simulink library "battery_monitor_lib"  (R2022b)
settings: Solver=VariableStepAuto  StartTime=0.0  StopTime=10.0  RelTol=1e-3
settings Model: Creator=dr_pa  LastModifiedBy=LinF

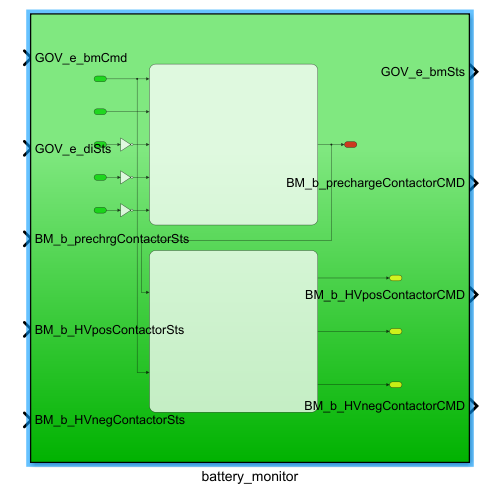
[thumbnail: Simulink's stored preview of the top-level diagram]
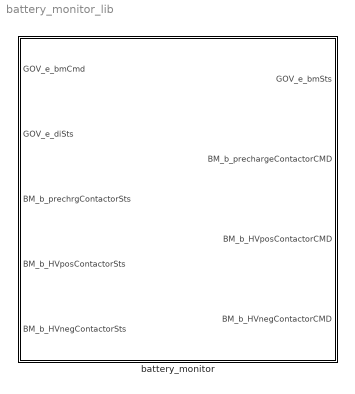
== system battery_monitor_lib ==
  battery_monitor : Subsystem
      settings: LibrarySourceBlock=battery_monitor_lib/battery_monitor

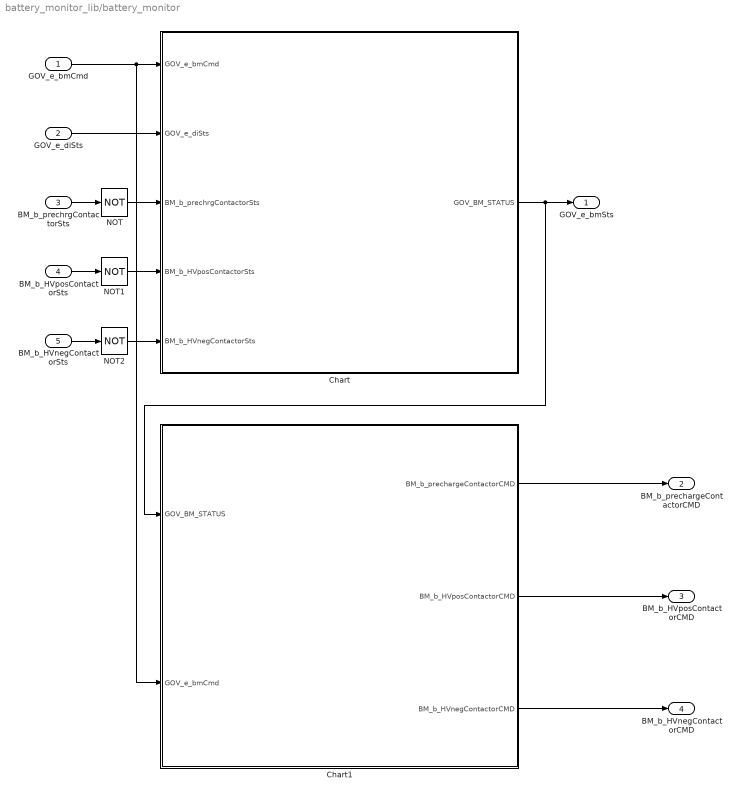
== system battery_monitor_lib/battery_monitor ==
  GOV_e_bmCmd : Inport
  GOV_e_diSts : Inport  Port=2
  BM_b_prechrgContactorSts : Inport  Port=3
  BM_b_HVposContactorSts : Inport  Port=4
  BM_b_HVnegContactorSts : Inport  Port=5
  Chart : Stateflow chart  TreatAsAtomicUnit=on
  Chart1 : Stateflow chart  TreatAsAtomicUnit=on
  NOT : Logic  Operator=NOT  IconShape=distinctive  AllPortsSameDT=off  OutDataTypeStr=boolean
  NOT1 : Logic  Operator=NOT  IconShape=distinctive  AllPortsSameDT=off  OutDataTypeStr=boolean
  NOT2 : Logic  Operator=NOT  IconShape=distinctive  AllPortsSameDT=off  OutDataTypeStr=boolean
  GOV_e_bmSts : Outport
  BM_b_prechargeContactorCMD : Outport  Port=2
  BM_b_HVposContactorCMD : Outport  Port=3
  BM_b_HVnegContactorCMD : Outport  Port=4
  wires:
  GOV_e_bmCmd/1 -> Chart/1(GOV_e_bmCmd), Chart1/2(GOV_e_bmCmd)
  BM_b_prechrgContactorSts/1 -> NOT/1
  BM_b_HVposContactorSts/1 -> NOT1/1
  BM_b_HVnegContactorSts/1 -> NOT2/1
  Chart/1(GOV_BM_STATUS) -> Chart1/1(GOV_BM_STATUS), GOV_e_bmSts/1
  Chart1/2(BM_b_HVposContactorCMD) -> BM_b_HVposContactorCMD/1
  Chart1/1(BM_b_prechargeContactorCMD) -> BM_b_prechargeContactorCMD/1
  Chart1/3(BM_b_HVnegContactorCMD) -> BM_b_HVnegContactorCMD/1
  GOV_e_diSts/1 -> Chart/2(GOV_e_diSts)
  NOT/1 -> Chart/3(BM_b_prechrgContactorSts)
  NOT1/1 -> Chart/4(BM_b_HVposContactorSts)
  NOT2/1 -> Chart/5(BM_b_HVnegContactorSts)

== stateflow chart battery_monitor_lib/battery_monitor/Chart ==
  state ErrorPrechargeClosedState [commented out]
    entry:
    GOV_BM_STATUS = ERR_PRECHARGE_CLOSED;
  state InitialState
    entry:
    GOV_BM_STATUS = BM_INIT;
  state ErrorStartupState
    entry:
    GOV_BM_STATUS = ERR_STARTUP;
  state ErrorAllClosedState [commented out]
    entry:
    GOV_BM_STATUS = ERR_ALL_CLOSED;
  state ErrorHVPositive [commented out]
    entry:
    GOV_BM_STATUS = ERR_HV_POSITIVE;
  state StartupState1
    entry:
    GOV_BM_STATUS = BM_IDLE;
  state StartupState
    entry:
    GOV_BM_STATUS = BM_STARTUP;
  state InitializePrechargeState
    entry:
    GOV_BM_STATUS = INIT_PRECHARGE;
  state ErrorInitializePrechargeState [commented out]
    entry:
    GOV_BM_STATUS = ERR_INIT_PRECHARGE;
  state PrechargeState
    entry:
    GOV_BM_STATUS = PRECHARGE;
  state ErrorPrechargeState [commented out]
    entry:
    GOV_BM_STATUS = ERR_PRECHARGE;
  state RunningState
    entry:
    GOV_BM_STATUS = BM_RUNNING;
  (default) -> InitialState
  InitialState -> ErrorStartupState [order 1] : [BM_b_prechrgContactorSts == 1 && BM_b_HVnegContactorSts == 0 && BM_b_HVposContactorSts == 0]
  InitialState -> ErrorStartupState [order 2] : [BM_b_prechrgContactorSts == 1 && BM_b_HVnegContactorSts == 1 && BM_b_HVposContactorSts == 1]
  InitialState -> ErrorStartupState [order 3] : [BM_b_prechrgContactorSts == 0 && BM_b_HVnegContactorSts == 0 && BM_b_HVposContactorSts == 1]
  RunningState -> InitialState [order 1] : [GOV_e_bmCmd == 1]
  InitialState -> StartupState1 [order 4] : [BM_b_prechrgContactorSts == 0 && BM_b_HVnegContactorSts == 0 && BM_b_HVposContactorSts == 0 && GOV_e_diSts == DI_STATUSES.DRV_START_REQ]
  StartupState -> ErrorStartupState [order 2] : after(100,sec)
  PrechargeState -> ErrorStartupState [order 2] : after(100,sec)
  InitializePrechargeState -> ErrorStartupState [order 2] : after(100,sec)
  StartupState1 -> StartupState : [BM_b_prechrgContactorSts == 0 && BM_b_HVnegContactorSts == 1 && BM_b_HVposContactorSts == 0]
  StartupState -> InitializePrechargeState [order 1] : [BM_b_prechrgContactorSts == 1 && BM_b_HVnegContactorSts == 1 && BM_b_HVposContactorSts == 0]
  InitializePrechargeState -> PrechargeState [order 1] : [BM_b_prechrgContactorSts == 1 && BM_b_HVnegContactorSts == 1 && BM_b_HVposContactorSts == 1]
  PrechargeState -> RunningState [order 1] : [BM_b_prechrgContactorSts == 0 && BM_b_HVnegContactorSts == 1 && BM_b_HVposContactorSts == 1]
  RunningState -> RunningState [order 2] : [BM_b_prechrgContactorSts == 0 && BM_b_HVnegContactorSts == 1 && BM_b_HVposContactorSts == 1]
  data: GOV_e_bmCmd input; GOV_e_diSts input; BM_b_prechrgContactorSts input; BM_b_HVposContactorSts input; BM_b_HVnegContactorSts input; GOV_BM_STATUS output Enum: BM_STATUSES

== stateflow chart battery_monitor_lib/battery_monitor/Chart1 ==
  state StartupCMD
    en:
    BM_b_prechargeContactorCMD = 0;
    BM_b_HVnegContactorCMD = 0;
    BM_b_HVposContactorCMD = 0;
  state Close_HVneg1
    en:
    BM_b_prechargeContactorCMD = 0;
    BM_b_HVnegContactorCMD = 1;
    BM_b_HVposContactorCMD = 0;
  state Close_precharge
    en:
    BM_b_prechargeContactorCMD = 1;
    BM_b_HVnegContactorCMD = 1;
    BM_b_HVposContactorCMD = 0;
  state Close_HVpos
    en:
    BM_b_prechargeContactorCMD = 1;
    BM_b_HVnegContactorCMD = 1;
    BM_b_HVposContactorCMD = 1;
  state Open_precharge
    en, du:
    BM_b_prechargeContactorCMD = 0;
    BM_b_HVnegContactorCMD = 1;
    BM_b_HVposContactorCMD = 1;
  (default) -> StartupCMD
  Open_precharge -> StartupCMD [order 2] : [GOV_e_bmCmd == 1]
  StartupCMD -> Close_HVneg1 : [GOV_BM_STATUS == BM_STATUSES.BM_IDLE]
  Close_HVneg1 -> Close_precharge : after(100,msec)[GOV_BM_STATUS == BM_STATUSES.BM_STARTUP]
  Close_precharge -> Close_HVpos : after(6500,msec)[GOV_BM_STATUS == BM_STATUSES.INIT_PRECHARGE]
  Close_HVpos -> Open_precharge : after(100,msec)[GOV_BM_STATUS == BM_STATUSES.PRECHARGE]
  Open_precharge -> Open_precharge [order 1] : [GOV_BM_STATUS == BM_STATUSES.BM_RUNNING]
  data: BM_b_prechargeContactorCMD output; BM_b_HVposContactorCMD output; BM_b_HVnegContactorCMD output; GOV_BM_STATUS input; GOV_e_bmCmd input
